simulink model "DrivetrainHevP4"  (R2023b)
settings: Solver=VariableStepAuto  StartTime=0.0  StopTime=inf  RelTol=1e-3  EnableMultiTasking=on
model workspace (MAT data in the model file):
  Aeff : Simulink.Parameter (value not decoded)
  Af : Simulink.Parameter (value not decoded)
  Bx : Simulink.Parameter (value not decoded)
  Cd : Simulink.Parameter (value not decoded)
  Cl : Simulink.Parameter (value not decoded)
  Cpm : Simulink.Parameter (value not decoded)
  Cx : Simulink.Parameter (value not decoded)
  Dx : Simulink.Parameter (value not decoded)
  Ex : Simulink.Parameter (value not decoded)
  FZMAX : Simulink.Parameter (value not decoded)
  FZMIN : Simulink.Parameter (value not decoded)
  Fc : Simulink.Parameter (value not decoded)
  FsbF : Simulink.Parameter (value not decoded)
  FsbR : Simulink.Parameter (value not decoded)
  FskF : Simulink.Parameter (value not decoded)
  FskR : Simulink.Parameter (value not decoded)
  G : Simulink.Parameter (value not decoded)
  G_o : Simulink.Parameter (value not decoded)
  Iyy : Simulink.Parameter (value not decoded)
  Iyy_Whl : Simulink.Parameter (value not decoded)
  J : Simulink.Parameter (value not decoded)
  J1 : Simulink.Parameter (value not decoded)
  J2 : Simulink.Parameter (value not decoded)
  Jd : Simulink.Parameter (value not decoded)
  Ji : Simulink.Parameter (value not decoded)
  Jin : Simulink.Parameter (value not decoded)
  Jin_Cltch : Simulink.Parameter (value not decoded)
  Jin_Cltch2 : Simulink.Parameter (value not decoded)
  Jout : Simulink.Parameter (value not decoded)
  Jout_Cltch : Simulink.Parameter (value not decoded)
  Jout_Cltch2 : Simulink.Parameter (value not decoded)
  Jt : Simulink.Parameter (value not decoded)
  Jw1 : Simulink.Parameter (value not decoded)
  Jw2 : Simulink.Parameter (value not decoded)
  K_c : Simulink.Parameter (value not decoded)
  Lrel : Simulink.Parameter (value not decoded)
  Mass : Simulink.Parameter (value not decoded)
  N : Simulink.Parameter (value not decoded)
  NF : Simulink.Parameter (value not decoded)
  NR : Simulink.Parameter (value not decoded)
  N_P4 : Simulink.Parameter (value not decoded)
  Ndiff : Simulink.Parameter (value not decoded)
  Ndiff_P4 : Simulink.Parameter (value not decoded)
  Ndisk : Simulink.Parameter (value not decoded)
  Ndisks : Simulink.Parameter (value not decoded)
  Pabs : Simulink.Parameter (value not decoded)
  Press : Simulink.Parameter (value not decoded)
  Re : Simulink.Parameter (value not decoded)
  Reff : Simulink.Parameter (value not decoded)
  Reff_LSD : Simulink.Parameter (value not decoded)
  Rm : Simulink.Parameter (value not decoded)
  T : Simulink.Parameter (value not decoded)
  Temp_bpts : Simulink.Parameter (value not decoded)
  Trq_bpts : Simulink.Parameter (value not decoded)
  UNLOADED_RADIUS : Simulink.Parameter (value not decoded)
  VXLOW : Simulink.Parameter (value not decoded)
  aMy : Simulink.Parameter (value not decoded)
  a_CG : Simulink.Parameter (value not decoded)
  alphaMy : Simulink.Parameter (value not decoded)
  b : Simulink.Parameter (value not decoded)
  b1 : Simulink.Parameter (value not decoded)
  b1_g : Simulink.Parameter (value not decoded)
  b2 : Simulink.Parameter (value not decoded)
  b2_g : Simulink.Parameter (value not decoded)
  bMy : Simulink.Parameter (value not decoded)
  b_CG : Simulink.Parameter (value not decoded)
  b_J : Simulink.Parameter (value not decoded)
  bd : Simulink.Parameter (value not decoded)
  betaMy : Simulink.Parameter (value not decoded)
  bi : Simulink.Parameter (value not decoded)
  bin : Simulink.Parameter (value not decoded)
  bin_Cltch : Simulink.Parameter (value not decoded)
  bout : Simulink.Parameter (value not decoded)
  bout_Cltch : Simulink.Parameter (value not decoded)
  br : Simulink.Parameter (value not decoded)
  bt : Simulink.Parameter (value not decoded)
  bw1 : Simulink.Parameter (value not decoded)
  bw2 : Simulink.Parameter (value not decoded)
  cMy : Simulink.Parameter (value not decoded)
  disk_abore : Simulink.Parameter (value not decoded)
  domega_o : Simulink.Parameter (value not decoded)
  dw : Simulink.Parameter (value not decoded)
  dzdotsF : Simulink.Parameter (value not decoded)
  dzdotsR : Simulink.Parameter (value not decoded)
  dzsF : Simulink.Parameter (value not decoded)
  dzsR : Simulink.Parameter (value not decoded)
  eta : Simulink.Parameter (value not decoded)
  eta_diff : Simulink.Parameter (value not decoded)
  eta_tbl : Simulink.Parameter (value not decoded)
  g : Simulink.Parameter (value not decoded)
  grEff : Simulink.Parameter (value not decoded)
  h : Simulink.Parameter (value not decoded)
  k : Simulink.Parameter (value not decoded)
  k1 : Simulink.Parameter (value not decoded)
  k2 : Simulink.Parameter (value not decoded)
  kappamax : Simulink.Parameter (value not decoded)
  lam_x : Simulink.Parameter (value not decoded)
  mu_kinetic : Simulink.Parameter (value not decoded)
  mu_static : Simulink.Parameter (value not decoded)
  muc : Simulink.Parameter (value not decoded)
  muk : Simulink.Parameter (value not decoded)
  mus : Simulink.Parameter (value not decoded)
  num_pads : Simulink.Parameter (value not decoded)
  omega1_c : Simulink.Parameter (value not decoded)
  omega2_c : Simulink.Parameter (value not decoded)
  omega_bpts : Simulink.Parameter (value not decoded)
  omega_c : Simulink.Parameter (value not decoded)
  omega_o : Simulink.Parameter (value not decoded)
  omega_o_J : Simulink.Parameter (value not decoded)
  omegai_o : Simulink.Parameter (value not decoded)
  omegain_o : Simulink.Parameter (value not decoded)
  omegal : Simulink.Parameter (value not decoded)
  omegao : Simulink.Parameter (value not decoded)
  omegaout_o : Simulink.Parameter (value not decoded)
  omegat_o : Simulink.Parameter (value not decoded)
  omegau : Simulink.Parameter (value not decoded)
  omegaw1o : Simulink.Parameter (value not decoded)
  omegaw2o : Simulink.Parameter (value not decoded)
  phi : Simulink.Parameter (value not decoded)
  philu : Simulink.Parameter (value not decoded)
  press : Simulink.Parameter (value not decoded)
  psi : Simulink.Parameter (value not decoded)
  q_o : Simulink.Parameter (value not decoded)
  tauC : Simulink.Parameter (value not decoded)
  tauC_1 : Simulink.Parameter (value not decoded)
  tauC_LSD : Simulink.Parameter (value not decoded)
  tauTC : Simulink.Parameter (value not decoded)
  tau_s : Simulink.Parameter (value not decoded)
  tc : Simulink.Parameter (value not decoded)
  theta_o : Simulink.Parameter (value not decoded)
  theta_o_Veh : Simulink.Parameter (value not decoded)
  ts : Simulink.Parameter (value not decoded)
  w1_o : Simulink.Parameter (value not decoded)
  wc : Simulink.Parameter (value not decoded)
  win_o : Simulink.Parameter (value not decoded)
  wout_o : Simulink.Parameter (value not decoded)
  x_o : Simulink.Parameter (value not decoded)
  xdot_o : Simulink.Parameter (value not decoded)
  z_o : Simulink.Parameter (value not decoded)
  zdot_o : Simulink.Parameter (value not decoded)
  zeta : Simulink.Parameter (value not decoded)
symbols that are objects in the model workspace (value not decoded): b, b_CG, g, k, Mass, N, T, Temp_bpts
undefined symbols (not defined in the file or in its folder): Lock, up
libraries: autolibsharedcoupling x4, autolibpowerinfoutils x4, autolibshared x3, autolibshareddiff x2, autolibutils x2, autolibsharedtransfixedgear x1, autolibtrqconv x1
(part 3 of 3)

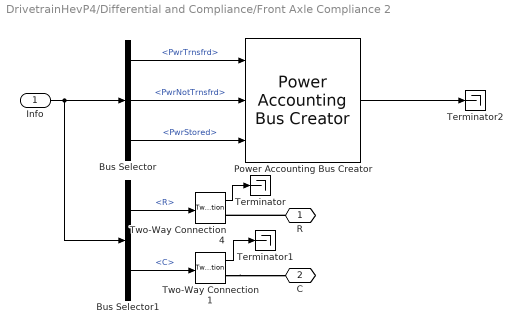
== system DrivetrainHevP4/Differential and Compliance/Front Axle Compliance 2 ==
  Info : Inport
  Bus Selector : BusSelector  OutputSignals=PwrInfo.PwrTrnsfrd,PwrInfo.PwrNotTrnsfrd,PwrInfo.PwrStored
  Bus Selector1 : BusSelector  OutputSignals=Trq.R,Trq.C
  Power Accounting Bus Creator : autolibpowerinfoutils/Power Accounting Bus Creator  AssctBlkSelPopup=Parent  RefBlkName='libraryname/blkname'  PwrTrnsfrdCheckBox=on  PwrNotTrnsfrdCheckBox=on  PwrStoredCheckBox=on  aMode=aMode
  Terminator : Terminator
  Terminator1 : Terminator
  Terminator2 : Terminator
  Two-Way Connection1 : TwoWayConnection
  Two-Way Connection4 : TwoWayConnection
  R : PMIOPort  Side=Left
  C : PMIOPort  Port=2  Side=Right
  wires:
  Bus Selector/3 -> Power Accounting Bus Creator/3  "<PwrStored>"
  Bus Selector/2 -> Power Accounting Bus Creator/2  "<PwrNotTrnsfrd>"
  Bus Selector/1 -> Power Accounting Bus Creator/1  "<PwrTrnsfrd>"
  Power Accounting Bus Creator/1 -> Terminator2/1
  Bus Selector1/2 -> Two-Way Connection1/1  "<C>"
  Bus Selector1/1 -> Two-Way Connection4/1  "<R>"
  Two-Way Connection1/1 -> Terminator1/1
  Info/1 -> Bus Selector/1, Bus Selector1/1
  Two-Way Connection4/1 -> Terminator/1
  connections:
  Two-Way Connection1/RConn1 -- C/RConn1
  R/RConn1 -- Two-Way Connection4/RConn1

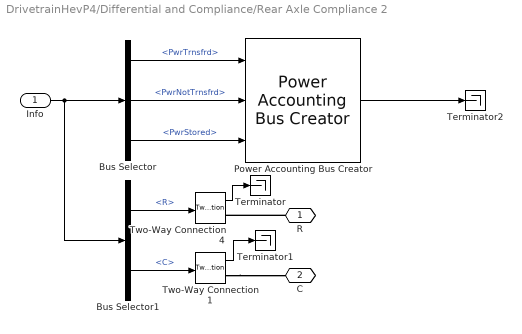
== system DrivetrainHevP4/Differential and Compliance/Rear Axle Compliance 2 ==
  Info : Inport
  Bus Selector : BusSelector  OutputSignals=PwrInfo.PwrTrnsfrd,PwrInfo.PwrNotTrnsfrd,PwrInfo.PwrStored
  Bus Selector1 : BusSelector  OutputSignals=Trq.R,Trq.C
  Power Accounting Bus Creator : autolibpowerinfoutils/Power Accounting Bus Creator  AssctBlkSelPopup=Parent  RefBlkName='libraryname/blkname'  PwrTrnsfrdCheckBox=on  PwrNotTrnsfrdCheckBox=on  PwrStoredCheckBox=on  aMode=aMode
  Terminator : Terminator
  Terminator1 : Terminator
  Terminator2 : Terminator
  Two-Way Connection1 : TwoWayConnection
  Two-Way Connection4 : TwoWayConnection
  R : PMIOPort  Side=Left
  C : PMIOPort  Port=2  Side=Right
  wires:
  Bus Selector/3 -> Power Accounting Bus Creator/3  "<PwrStored>"
  Bus Selector/2 -> Power Accounting Bus Creator/2  "<PwrNotTrnsfrd>"
  Bus Selector/1 -> Power Accounting Bus Creator/1  "<PwrTrnsfrd>"
  Power Accounting Bus Creator/1 -> Terminator2/1
  Bus Selector1/2 -> Two-Way Connection1/1  "<C>"
  Bus Selector1/1 -> Two-Way Connection4/1  "<R>"
  Two-Way Connection1/1 -> Terminator1/1
  Info/1 -> Bus Selector/1, Bus Selector1/1
  Two-Way Connection4/1 -> Terminator/1
  connections:
  Two-Way Connection1/RConn1 -- C/RConn1
  R/RConn1 -- Two-Way Connection4/RConn1

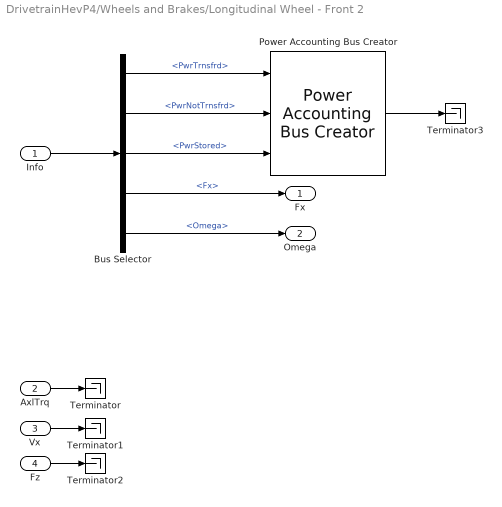
== system DrivetrainHevP4/Wheels and Brakes/Longitudinal Wheel - Front 2 ==
  Info : Inport
  AxlTrq : Inport  Port=2
  Vx : Inport  Port=3
  Fz : Inport  Port=4
  Bus Selector : BusSelector  OutputSignals=PwrInfo.PwrTrnsfrd,PwrInfo.PwrNotTrnsfrd,PwrInfo.PwrStored,Fx,Omega
  Power Accounting Bus Creator : autolibpowerinfoutils/Power Accounting Bus Creator  AssctBlkSelPopup=Parent  RefBlkName='libraryname/blkname'  PwrTrnsfrdCheckBox=on  PwrNotTrnsfrdCheckBox=on  PwrStoredCheckBox=on  aMode=aMode
  Terminator{,1..3} (4 alike) : Terminator
  Fx : Outport  VectorParamsAs1DForOutWhenUnconnected=off
  Omega : Outport  Port=2  VectorParamsAs1DForOutWhenUnconnected=off
  wires:
  Power Accounting Bus Creator/1 -> Terminator3/1
  Bus Selector/5 -> Omega/1  "<Omega>"
  Bus Selector/4 -> Fx/1  "<Fx>"
  Bus Selector/3 -> Power Accounting Bus Creator/3  "<PwrStored>"
  Bus Selector/2 -> Power Accounting Bus Creator/2  "<PwrNotTrnsfrd>"
  Bus Selector/1 -> Power Accounting Bus Creator/1  "<PwrTrnsfrd>"
  Info/1 -> Bus Selector/1
  Fz/1 -> Terminator2/1
  Vx/1 -> Terminator1/1
  AxlTrq/1 -> Terminator/1

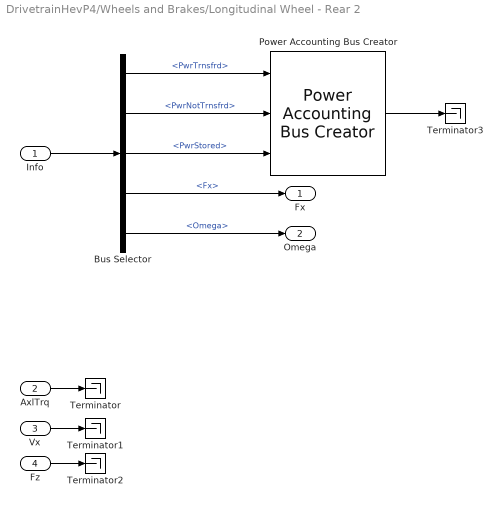
== system DrivetrainHevP4/Wheels and Brakes/Longitudinal Wheel - Rear 2 ==
  Info : Inport
  AxlTrq : Inport  Port=2
  Vx : Inport  Port=3
  Fz : Inport  Port=4
  Bus Selector : BusSelector  OutputSignals=PwrInfo.PwrTrnsfrd,PwrInfo.PwrNotTrnsfrd,PwrInfo.PwrStored,Fx,Omega
  Power Accounting Bus Creator : autolibpowerinfoutils/Power Accounting Bus Creator  AssctBlkSelPopup=Parent  RefBlkName='libraryname/blkname'  PwrTrnsfrdCheckBox=on  PwrNotTrnsfrdCheckBox=on  PwrStoredCheckBox=on  aMode=aMode
  Terminator{,1..3} (4 alike) : Terminator
  Fx : Outport  VectorParamsAs1DForOutWhenUnconnected=off
  Omega : Outport  Port=2  VectorParamsAs1DForOutWhenUnconnected=off
  wires:
  Power Accounting Bus Creator/1 -> Terminator3/1
  Bus Selector/5 -> Omega/1  "<Omega>"
  Bus Selector/4 -> Fx/1  "<Fx>"
  Bus Selector/3 -> Power Accounting Bus Creator/3  "<PwrStored>"
  Bus Selector/2 -> Power Accounting Bus Creator/2  "<PwrNotTrnsfrd>"
  Bus Selector/1 -> Power Accounting Bus Creator/1  "<PwrTrnsfrd>"
  Info/1 -> Bus Selector/1
  Fz/1 -> Terminator2/1
  Vx/1 -> Terminator1/1
  AxlTrq/1 -> Terminator/1
